simulink model "controle_02"  (R2014b)
settings: Solver=ode45  StartTime=0.0  StopTime=t_run  RelTol=1e-3
values from neighbouring files (symbols this model uses):
  den_G = G.den{:}    [sim_01.m]
  num_G = G.num{:}    [sim_01.m]
  t_step = 1    [sim_01.m]
  Ts = 0.01    [pid_custom.m]
undefined symbols (not defined in the file or in its folder): den_C_d, num_C_d
settings Model: Creator=PC  LastModifiedBy=PC

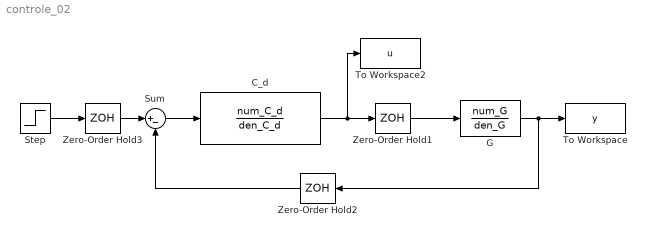
== system controle_02 ==
  C_d : DiscreteTransferFcn  Numerator=num_C_d  Denominator=den_C_d  SampleTime=Ts
  G : TransferFcn  Numerator=num_G  Denominator=den_G
  Step : Step  Time=t_step
  Sum : Sum  Inputs=|+-  SampleTime=Ts
  To Workspace : ToWorkspace  VariableName=y  SampleTime=-1
  To Workspace2 : ToWorkspace  VariableName=u  SampleTime=-1
  Zero-Order Hold1 : ZeroOrderHold  SampleTime=Ts
  Zero-Order Hold2 : ZeroOrderHold  SampleTime=Ts
  Zero-Order Hold3 : ZeroOrderHold  SampleTime=Ts
  wires:
  Step/1 -> Zero-Order Hold3/1
  Sum/1 -> C_d/1
  C_d/1 -> Zero-Order Hold1/1, To Workspace2/1
  Zero-Order Hold1/1 -> G/1
  Zero-Order Hold2/1 -> Sum/2
  Zero-Order Hold3/1 -> Sum/1
  G/1 -> To Workspace/1, Zero-Order Hold2/1
